simulink subsystem "GPS_MAX_M10S"  (R2025b)
settings: Solver=VariableStepAuto  StartTime=0.0  StopTime=10.0  RelTol=1e-3
undefined symbols (not defined in the file): gps_converter
settings Model: Creator=Admin  LastModifiedBy=slee7

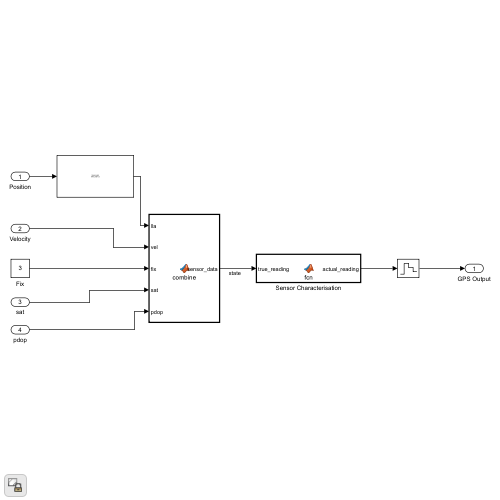
[thumbnail: Simulink's stored preview of the top-level diagram]
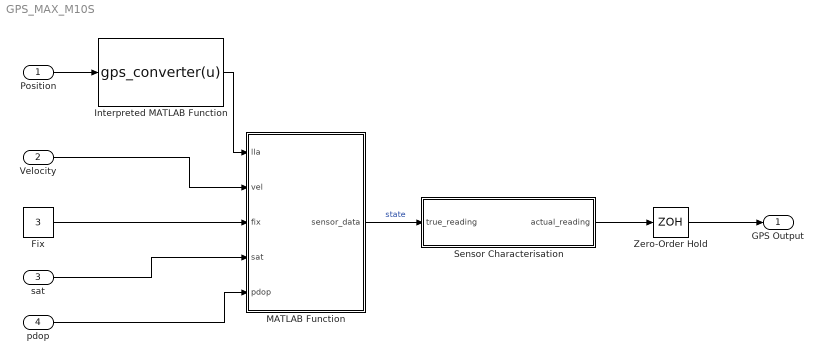
== system GPS_MAX_M10S ==
  Position : Inport
  Velocity : Inport  Port=2
  sat : Inport  Port=3
  pdop : Inport  Port=4
  Fix : Constant  Value=3
  Interpreted MATLAB Function : MATLABFcn  MATLABFcn=gps_converter(u)  OutputDimensions=[3 1]  Output1D=off
  MATLAB Function : MATLAB Function  TreatAsAtomicUnit=on
  Sensor Characterisation : MATLAB Function  TreatAsAtomicUnit=on
  Zero-Order Hold : ZeroOrderHold  SampleTime=0.1
  GPS Output : Outport
  wires:
  MATLAB Function/1(sensor_data) -> Sensor Characterisation/1(true_reading)  "state"
  Zero-Order Hold/1 -> GPS Output/1
  Sensor Characterisation/1(actual_reading) -> Zero-Order Hold/1
  Velocity/1 -> MATLAB Function/2(vel)
  Fix/1 -> MATLAB Function/3(fix)
  sat/1 -> MATLAB Function/4(sat)
  pdop/1 -> MATLAB Function/5(pdop)
  Position/1 -> Interpreted MATLAB Function/1
  Interpreted MATLAB Function/1 -> MATLAB Function/1(lla)

== matlab function GPS_MAX_M10S/MATLAB Function ==
  data: lla input; sensor_data output; vel input; fix input; sat input; pdop input
function sensor_data = combine(lla, vel, fix, sat, pdop)

sensor_data = [lla; vel; fix; sat; pdop];

end

== matlab function GPS_MAX_M10S/Sensor Characterisation ==
  data: true_reading input; actual_reading output
function actual_reading = fcn(true_reading)
%#codegen
    persistent b_previous

    % true_reading = [lat; lon; alt; v_n; v_e; v_d; fix; sat; pdop]
    dt = 0.02;   % 20 ms

    % Ensure column vector
    true_reading = true_reading(:);

    % Number of channels
    n = 9;

    % Initialise persistent drift state
    if isempty(b_previous)
        b_previous = zeros(n,1);
    end

    % -----------------------------
    % Constant bias
    % -----------------------------
    b_const = zeros(n,1);

    % -----------------------------
    % Drift bias (Gauss-Markov)
    % -----------------------------
    tau = [116.2031;   % lat
           204.0083;   % lon
            88.1618;   % alt
             0.3353;   % v_n
             1.4466;   % v_e
             0.8506;   % v_d
                inf;   % fix
                inf;   % sat
                inf];  % pdop

    q = [6.1178e-13;   % lat drift variance
         7.8958e-13;   % lon drift variance
         1.0101e+04;   % alt drift variance
         1.1742e+02;   % v_n drift variance
         6.3880e+01;   % v_e drift variance
         9.5787e+01;   % v_d drift variance
         0;            % fix
         0;            % sat
         0];           % pdop

    omega = sqrt(q) .* randn(n,1);
    b_drift = exp(-dt ./ tau) .* b_previous + omega;

    composite_bias = b_const + b_drift;

    % Update persistent state
    b_previous = b_drift;

    % -----------------------------
    % Gaussian noise
    % -----------------------------
    noise_std = [1.35e-05;   % lat
                 1.35e-05;   % lon
                 1.35e-05;   % alt
                 0.05;       % v_n
                 0.05;       % v_e
                 0.05;       % v_d
                 0;          % fix
                 0;          % sat
                 0];         % pdop

    noise = noise_std .* randn(n,1);

    % -----------------------------
    % Quantisation
    % -----------------------------
    quant_step = [0.5;  % lat
                  0.5;  % lon
                  0.5;  % alt
                  0.5;  % v_n
                  0.5;  % v_e
                  0.5;  % v_d
                  1;    % fix
                  1;    % sat
                  0.1]; % pdop

    % -----------------------------
    % Reading processing
    % -----------------------------
    actual_reading_continuous = true_reading + composite_bias + noise;
    actual_reading = quant_step .* round(actual_reading_continuous ./ quant_step);

    % -----------------------------
    % Post-processing discrete fields
    % -----------------------------
    % fix should be integer and non-negative
    actual_reading(7) = max(0, round(actual_reading(7)));

    % sat should be integer and non-negative
    actual_reading(8) = max(0, round(actual_reading(8)));

    % pdop should not be negative
    actual_reading(9) = max(0, actual_reading(9));
end
